simulink model "PIDController"  (R2025b)
settings: Solver=VariableStepAuto  StartTime=0.0  StopTime=10.0  RelTol=1e-3

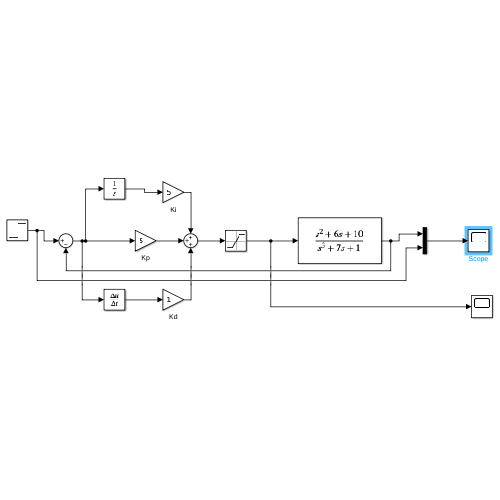
[thumbnail: Simulink's stored preview of the top-level diagram]
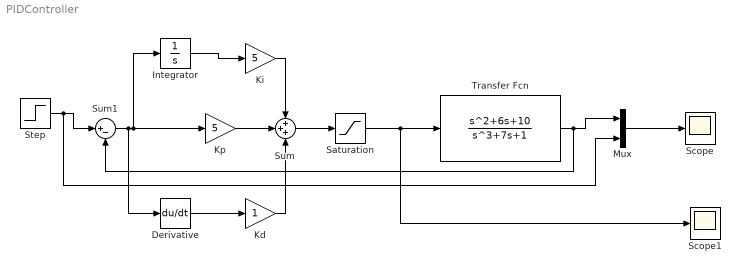
== system PIDController ==
  Derivative : Derivative
  Integrator : Integrator
  Kd : Gain
  Ki : Gain  Gain=5
  Kp : Gain  Gain=5
  Mux : Mux  Inputs=2
  Saturation : Saturate  UpperLimit=2  LowerLimit=-2
  Scope : Scope
      settings: ActiveDisplayYMinimum=-0.14155789594529691  ActiveDisplayYMaximum=1.2740210635076725
  Scope1 : Scope
  Step : Step  SampleTime=0
  Sum : Sum  Inputs=+++
  Sum1 : Sum  Inputs=|+-
  Transfer Fcn : TransferFcn  Numerator=[1, 6, 10]  Denominator=[1 0 7 1]
  wires:
  Step/1 -> Mux/2, Sum1/1
  Kp/1 -> Sum/2
  Sum1/1 -> Derivative/1, Integrator/1, Kp/1
  Integrator/1 -> Ki/1
  Derivative/1 -> Kd/1
  Ki/1 -> Sum/1
  Kd/1 -> Sum/3
  Saturation/1 -> Scope1/1, Transfer Fcn/1
  Sum/1 -> Saturation/1
  Transfer Fcn/1 -> Sum1/2, Mux/1
  Mux/1 -> Scope/1
